simulink model "SteeringWheel"  (R2024b)
settings: configuration reference "STM32H7_Config" (kept outside this file)
libraries: simulink x3
(part 1 of 2)
settings Model: DataDictionary=Master_Dictionary.sldd  EnableAccessToBaseWorkspace=off  Creator=torni  LastModifiedBy=Will
settings ConfigSetRef: SourceName=STM32H7_Config

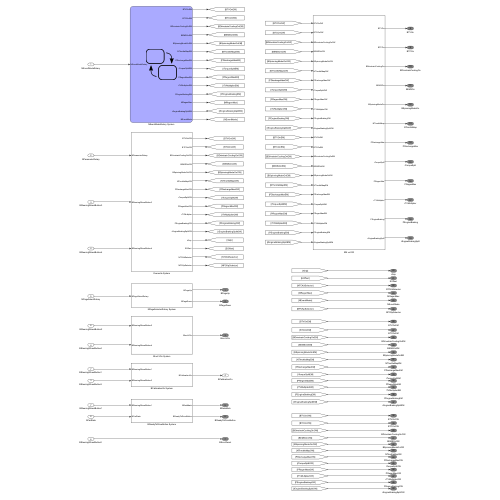
[thumbnail: Simulink's stored preview of the top-level diagram]
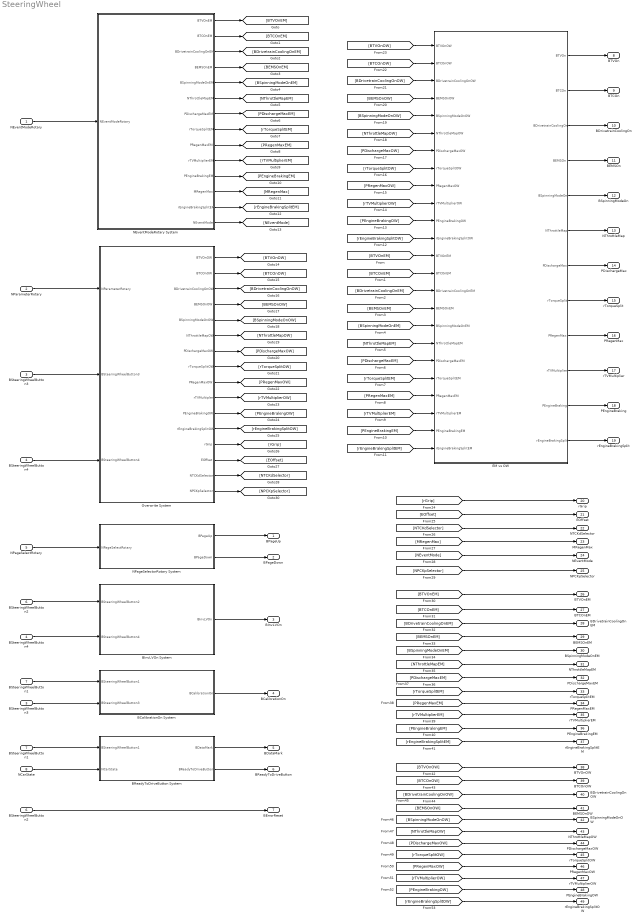
== system SteeringWheel ==
  NEventModeRotary : Inport
  NParameterRotary : Inport  Port=2
  BSteeringWheelButton3 : Inport  Port=3  OutDataTypeStr=boolean
  BSteeringWheelButton4 : Inport  Port=4  OutDataTypeStr=boolean
  NPageSelectRotary : Inport  Port=5
  BSteeringWheelButton2 : Inport  Port=6
  "BSteeringWheelButton1 " : Inport  Port=7
  NCarState : Inport  Port=8
  BCalibrationOn System : Subsystem
  BInvLVOn System : Subsystem
  BReadyToDriveButton System : Subsystem
  BSteeringWheelButton1 : InportShadow  Port=7
  "BSteeringWheelButton2 " : InportShadow  Port=6
  "BSteeringWheelButton3 " : InportShadow  Port=3  OutDataTypeStr=boolean
  "BSteeringWheelButton4 " : InportShadow  Port=4  OutDataTypeStr=boolean
  EM vs OW : Subsystem
  NEventModeRotary System : Stateflow chart  TreatAsAtomicUnit=on
  NPageSelectorRotary System : Subsystem
  Overwrite System : Subsystem
  BPageUp : Outport  VectorParamsAs1DForOutWhenUnconnected=off
  BPageDown : Outport  Port=2  VectorParamsAs1DForOutWhenUnconnected=off
  BInvLVOn : Outport  Port=3  VectorParamsAs1DForOutWhenUnconnected=off
  BCalibrationOn : Outport  Port=4  VectorParamsAs1DForOutWhenUnconnected=off
  BDataMark : Outport  Port=5  VectorParamsAs1DForOutWhenUnconnected=off
  BReadyToDriveButton : Outport  Port=6  VectorParamsAs1DForOutWhenUnconnected=off
  BErrorReset : Outport  Port=7  VectorParamsAs1DForOutWhenUnconnected=off
  BTVOn : Outport  Port=8  VectorParamsAs1DForOutWhenUnconnected=off
  BTCOn : Outport  Port=9  VectorParamsAs1DForOutWhenUnconnected=off
  BDrivetrainCoolingOn : Outport  Port=10  VectorParamsAs1DForOutWhenUnconnected=off
  BEMSOn : Outport  Port=11  VectorParamsAs1DForOutWhenUnconnected=off
  BSpinningModeOn : Outport  Port=12  VectorParamsAs1DForOutWhenUnconnected=off
  NThrottleMap : Outport  Port=13  VectorParamsAs1DForOutWhenUnconnected=off
  PDischargeMax : Outport  Port=14  VectorParamsAs1DForOutWhenUnconnected=off
  rTorqueSplit : Outport  Port=15  VectorParamsAs1DForOutWhenUnconnected=off
  PRegenMax : Outport  Port=16  VectorParamsAs1DForOutWhenUnconnected=off
  rTVMultiplier : Outport  Port=17  VectorParamsAs1DForOutWhenUnconnected=off
  PEngineBraking : Outport  Port=18  VectorParamsAs1DForOutWhenUnconnected=off
  rEngineBrakingSplit : Outport  Port=19  VectorParamsAs1DForOutWhenUnconnected=off
  rGrip : Outport  Port=20  VectorParamsAs1DForOutWhenUnconnected=off
  EOffset : Outport  Port=21  VectorParamsAs1DForOutWhenUnconnected=off
  NTCKdSelector : Outport  Port=22  VectorParamsAs1DForOutWhenUnconnected=off
  MRegenMax : Outport  Port=23  VectorParamsAs1DForOutWhenUnconnected=off
  NEventMode : Outport  Port=24  VectorParamsAs1DForOutWhenUnconnected=off
  NPCKpSelector : Outport  Port=25  VectorParamsAs1DForOutWhenUnconnected=off
  BTVOnEM : Outport  Port=26  OutDataTypeStr=double  VectorParamsAs1DForOutWhenUnconnected=off
  BTCOnEM : Outport  Port=27  OutDataTypeStr=double  VectorParamsAs1DForOutWhenUnconnected=off
  BDrivetrainCoolingOnEM : Outport  Port=28  OutDataTypeStr=double  VectorParamsAs1DForOutWhenUnconnected=off
  BEMSOnEM : Outport  Port=29  OutDataTypeStr=double  VectorParamsAs1DForOutWhenUnconnected=off
  BSpinningModeOnEM : Outport  Port=30  OutDataTypeStr=double  VectorParamsAs1DForOutWhenUnconnected=off
  NThrottleMapEM : Outport  Port=31  OutDataTypeStr=double  VectorParamsAs1DForOutWhenUnconnected=off
  PDischargeMaxEM : Outport  Port=32  OutDataTypeStr=double  VectorParamsAs1DForOutWhenUnconnected=off
  rTorqueSplitEM : Outport  Port=33  OutDataTypeStr=double  VectorParamsAs1DForOutWhenUnconnected=off
  PRegenMaxEM : Outport  Port=34  OutDataTypeStr=double  VectorParamsAs1DForOutWhenUnconnected=off
  rTVMultiplierEM : Outport  Port=35  OutDataTypeStr=double  VectorParamsAs1DForOutWhenUnconnected=off
  PEngineBrakingEM : Outport  Port=36  OutDataTypeStr=double  VectorParamsAs1DForOutWhenUnconnected=off
  rEngineBrakingSplitEM : Outport  Port=37  OutDataTypeStr=double  VectorParamsAs1DForOutWhenUnconnected=off
  BTVOnOW : Outport  Port=38  OutDataTypeStr=double  VectorParamsAs1DForOutWhenUnconnected=off
  BTCOnOW : Outport  Port=39  OutDataTypeStr=double  VectorParamsAs1DForOutWhenUnconnected=off
  BDrivetrainCoolingOnOW : Outport  Port=40  OutDataTypeStr=double  VectorParamsAs1DForOutWhenUnconnected=off
  BEMSOnOW : Outport  Port=41  OutDataTypeStr=double  VectorParamsAs1DForOutWhenUnconnected=off
  BSpinningModeOnOW : Outport  Port=42  OutDataTypeStr=double  VectorParamsAs1DForOutWhenUnconnected=off
  NThrottleMapOW : Outport  Port=43  OutDataTypeStr=double  VectorParamsAs1DForOutWhenUnconnected=off
  PDischargeMaxOW : Outport  Port=44  OutDataTypeStr=double  VectorParamsAs1DForOutWhenUnconnected=off
  rTorqueSplitOW : Outport  Port=45  OutDataTypeStr=double  VectorParamsAs1DForOutWhenUnconnected=off
  PRegenMaxOW : Outport  Port=46  OutDataTypeStr=double  VectorParamsAs1DForOutWhenUnconnected=off
  rTVMultiplierOW : Outport  Port=47  OutDataTypeStr=double  VectorParamsAs1DForOutWhenUnconnected=off
  PEngineBrakingOW : Outport  Port=48  OutDataTypeStr=double  VectorParamsAs1DForOutWhenUnconnected=off
  rEngineBrakingSplitOW : Outport  Port=49  OutDataTypeStr=double  VectorParamsAs1DForOutWhenUnconnected=off
  wires:
  BSteeringWheelButton3/1 -> Overwrite System/2(BSteeringWheelButton3)
  BSteeringWheelButton4/1 -> Overwrite System/3(BSteeringWheelButton4)
  [rEngineBrakingSplitOW] -> rEngineBrakingSplitOW/1
  [PEngineBrakingOW] -> PEngineBrakingOW/1
  [rTVMultiplierOW] -> rTVMultiplierOW/1
  [PRegenMaxOW] -> PRegenMaxOW/1
  [rTorqueSplitOW] -> rTorqueSplitOW/1
  [PDischargeMaxOW] -> PDischargeMaxOW/1
  [NThrottleMapOW] -> NThrottleMapOW/1
  [BSpinningModeOnOW] -> BSpinningModeOnOW/1
  [BEMSOnOW] -> BEMSOnOW/1
  [BDrivetrainCoolingOnOW] -> BDrivetrainCoolingOnOW/1
  [BTCOnOW] -> BTCOnOW/1
  [BTVOnOW] -> BTVOnOW/1
  [rEngineBrakingSplitEM] -> rEngineBrakingSplitEM/1
  [PEngineBrakingEM] -> PEngineBrakingEM/1
  [rTVMultiplierEM] -> rTVMultiplierEM/1
  [PRegenMaxEM] -> PRegenMaxEM/1
  [rTorqueSplitEM] -> rTorqueSplitEM/1
  [PDischargeMaxEM] -> PDischargeMaxEM/1
  [NThrottleMapEM] -> NThrottleMapEM/1
  [BSpinningModeOnEM] -> BSpinningModeOnEM/1
  [BEMSOnEM] -> BEMSOnEM/1
  [BDrivetrainCoolingOnEM] -> BDrivetrainCoolingOnEM/1
  [BTCOnEM] -> BTCOnEM/1
  [BTVOnEM] -> BTVOnEM/1
  [NPCKpSelector] -> NPCKpSelector/1
  [NEventMode] -> NEventMode/1
  [MRegenMax] -> MRegenMax/1
  [NTCKdSelector] -> NTCKdSelector/1
  [EOffset] -> EOffset/1
  [rGrip] -> rGrip/1
  EM vs OW/12(rEngineBrakingSplit) -> rEngineBrakingSplit/1
  EM vs OW/11(PEngineBraking) -> PEngineBraking/1
  EM vs OW/10(rTVMultiplier) -> rTVMultiplier/1
  EM vs OW/9(PRegenMax) -> PRegenMax/1
  EM vs OW/8(rTorqueSplit) -> rTorqueSplit/1
  EM vs OW/7(PDischargeMax) -> PDischargeMax/1
  EM vs OW/6(NThrottleMap) -> NThrottleMap/1
  EM vs OW/5(BSpinningModeOn) -> BSpinningModeOn/1
  EM vs OW/4(BEMSOn) -> BEMSOn/1
  EM vs OW/3(BDrivetrainCoolingOn) -> BDrivetrainCoolingOn/1
  EM vs OW/2(BTCOn) -> BTCOn/1
  EM vs OW/1(BTVOn) -> BTVOn/1
  NEventModeRotary System/14(NEventMode) -> [NEventMode]
  NEventModeRotary System/13(rEngineBrakingSplitEM) -> [rEngineBrakingSplitEM]
  NEventModeRotary System/12(MRegenMax) -> [MRegenMax]
  NEventModeRotary System/11(PEngineBrakingEM) -> [PEngineBrakingEM]
  NEventModeRotary System/10(rTVMultiplierEM) -> [rTVMultiplierEM]
  NEventModeRotary System/9(PRegenMaxEM) -> [PRegenMaxEM]
  NEventModeRotary System/8(rTorqueSplitEM) -> [rTorqueSplitEM]
  NEventModeRotary System/7(PDischargeMaxEM) -> [PDischargeMaxEM]
  NEventModeRotary System/6(NThrottleMapEM) -> [NThrottleMapEM]
  NEventModeRotary System/5(BSpinningModeOnEM) -> [BSpinningModeOnEM]
  NEventModeRotary System/4(BEMSOnEM) -> [BEMSOnEM]
  NEventModeRotary System/3(BDrivetrainCoolingOnEM) -> [BDrivetrainCoolingOnEM]
  NEventModeRotary System/2(BTCOnEM) -> [BTCOnEM]
  NEventModeRotary System/1(BTVOnEM) -> [BTVOnEM]
  NEventModeRotary/1 -> NEventModeRotary System/1(NEventModeRotary)
  Overwrite System/15(NTCKdSelector) -> [NTCKdSelector]
  Overwrite System/14("EOffset ") -> [EOffset]
  Overwrite System/13("rGrip ") -> [rGrip]
  Overwrite System/12(rEngineBrakingSplitOW) -> [rEngineBrakingSplitOW]
  Overwrite System/11(PEngineBrakingOW) -> [PEngineBrakingOW]
  Overwrite System/10(rTVMultipler) -> [rTVMultiplierOW]
  Overwrite System/9(PRegenMaxOW) -> [PRegenMaxOW]
  Overwrite System/8(rTorqueSplitOW) -> [rTorqueSplitOW]
  Overwrite System/7(PDischargeMaxOW) -> [PDischargeMaxOW]
  Overwrite System/6(NThrottleMapOW) -> [NThrottleMapOW]
  Overwrite System/5(BSpinningModeOnOW) -> [BSpinningModeOnOW]
  Overwrite System/4(BEMSOnOW) -> [BEMSOnOW]
  Overwrite System/3(BDrivetrainCoolingOnOW) -> [BDrivetrainCoolingOnOW]
  Overwrite System/2(BTCOnOW) -> [BTCOnOW]
  Overwrite System/1(BTVOnOW) -> [BTVOnOW]
  Overwrite System/16(NPCKpSelector) -> [NPCKpSelector]
  NParameterRotary/1 -> Overwrite System/1(NParameterRotary)
  NPageSelectRotary/1 -> NPageSelectorRotary System/1(NPageSelectRotary)
  NPageSelectorRotary System/1(BPageUp) -> BPageUp/1
  NPageSelectorRotary System/2(BPageDown) -> BPageDown/1
  BSteeringWheelButton2/1 -> BInvLVOn System/1(BSteeringWheelButton2)
  "BSteeringWheelButton4 "/1 -> BInvLVOn System/2(BSteeringWheelButton4)
  BInvLVOn System/1(BInvLVOn) -> BInvLVOn/1
  "BSteeringWheelButton1 "/1 -> BCalibrationOn System/1(BSteeringWheelButton1)
  "BSteeringWheelButton3 "/1 -> BCalibrationOn System/2("BSteeringWheelButton3 ")
  BCalibrationOn System/1(BCalibrationOn) -> BCalibrationOn/1
  BReadyToDriveButton System/1(BDataMark) -> BDataMark/1
  BReadyToDriveButton System/2(BReadyToDriveButton) -> BReadyToDriveButton/1
  BSteeringWheelButton1/1 -> BReadyToDriveButton System/1(BSteeringWheelButton1)
  NCarState/1 -> BReadyToDriveButton System/2(NCarState)
  "BSteeringWheelButton2 "/1 -> BErrorReset/1
  [BTVOnOW] -> EM vs OW/1(BTVOnOW)
  [BTCOnOW] -> EM vs OW/2(BTCOnOW)
  [BDrivetrainCoolingOnOW] -> EM vs OW/3(BDrivetrainCoolingOnOW)
  [BEMSOnOW] -> EM vs OW/4(BEMSOnOW)
  [BSpinningModeOnOW] -> EM vs OW/5(BSpinningModeOnOW)
  [NThrottleMapOW] -> EM vs OW/6(NThrottleMapOW)
  [PDischargeMaxOW] -> EM vs OW/7(PDischargeMaxOW)
  [rTorqueSplitOW] -> EM vs OW/8(rTorqueSplitOW)
  [PRegenMaxOW] -> EM vs OW/9(PRegenMaxOW)
  [rTVMultiplierOW] -> EM vs OW/10(rTVMultiplierOW)
  [PEngineBrakingOW] -> EM vs OW/11(PEngineBrakingOW)
  [rEngineBrakingSplitOW] -> EM vs OW/12(rEngineBrakingSplitOW)
  [BTVOnEM] -> EM vs OW/13(BTVOnEM)
  [BTCOnEM] -> EM vs OW/14(BTCOnEM)
  [BDrivetrainCoolingOnEM] -> EM vs OW/15(BDrivetrainCoolingOnEM)
  [BEMSOnEM] -> EM vs OW/16(BEMSOnEM)
  [BSpinningModeOnEM] -> EM vs OW/17(BSpinningModeOnEM)
  [NThrottleMapEM] -> EM vs OW/18(NThrottleMapEM)
  [PDischargeMaxEM] -> EM vs OW/19(PDischargeMaxEM)
  [rTorqueSplitEM] -> EM vs OW/20(rTorqueSplitEM)
  [PRegenMaxEM] -> EM vs OW/21(PRegenMaxEM)
  [rTVMultiplierEM] -> EM vs OW/22(rTVMultiplierEM)
  [PEngineBrakingEM] -> EM vs OW/23(PEngineBrakingEM)
  [rEngineBrakingSplitEM] -> EM vs OW/24(rEngineBrakingSplitEM)

== system SteeringWheel/BCalibrationOn System ==
  BSteeringWheelButton1 : Inport
  "BSteeringWheelButton3 " : Inport  Port=2
  AND : Logic  AllPortsSameDT=off  OutDataTypeStr=boolean
  BCalibrationOn : Outport  VectorParamsAs1DForOutWhenUnconnected=off
  wires:
  BSteeringWheelButton1/1 -> AND/1
  AND/1 -> BCalibrationOn/1
  "BSteeringWheelButton3 "/1 -> AND/2

== system SteeringWheel/BInvLVOn System ==
  BSteeringWheelButton2 : Inport
  BSteeringWheelButton4 : Inport  Port=2
  AND1 : Logic  Operator=NAND  AllPortsSameDT=off  OutDataTypeStr=boolean
  BInvLVOn : Outport  VectorParamsAs1DForOutWhenUnconnected=off
  wires:
  AND1/1 -> BInvLVOn/1
  BSteeringWheelButton2/1 -> AND1/1
  BSteeringWheelButton4/1 -> AND1/2

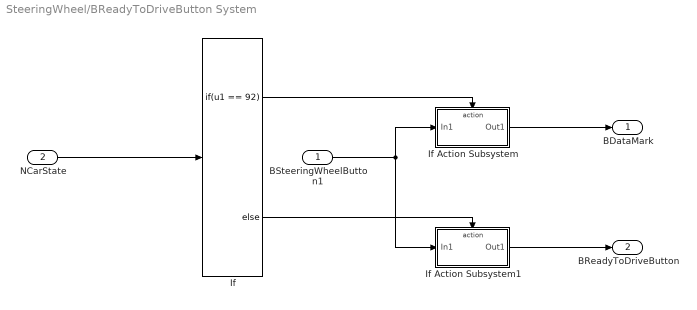
== system SteeringWheel/BReadyToDriveButton System ==
  BSteeringWheelButton1 : Inport
  NCarState : Inport  Port=2
  If : If  IfExpression=u1 == 92
  If Action Subsystem : Subsystem  TreatAsAtomicUnit=on
  If Action Subsystem1 : Subsystem  TreatAsAtomicUnit=on
  BDataMark : Outport  VectorParamsAs1DForOutWhenUnconnected=off
  BReadyToDriveButton : Outport  Port=2  VectorParamsAs1DForOutWhenUnconnected=off
  wires:
  If/2 -> If Action Subsystem1/Action
  If Action Subsystem/1(Out1) -> BDataMark/1
  If Action Subsystem1/1(Out1) -> BReadyToDriveButton/1
  BSteeringWheelButton1/1 -> If Action Subsystem1/1(In1), If Action Subsystem/1(In1)
  NCarState/1 -> If/1
  If/1 -> If Action Subsystem/Action

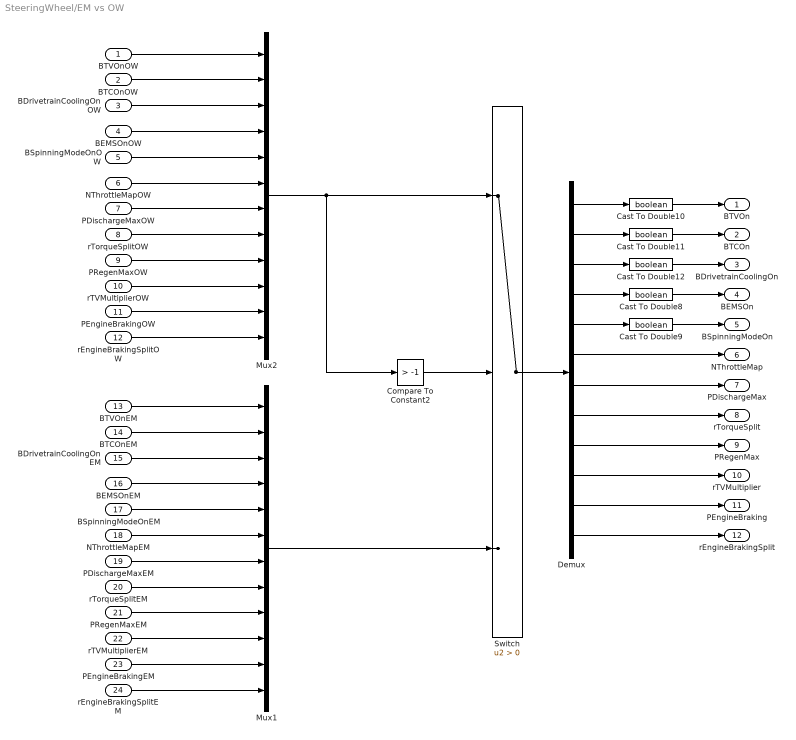
== system SteeringWheel/EM vs OW ==
  BTVOnOW : Inport
  BTCOnOW : Inport  Port=2
  BDrivetrainCoolingOnOW : Inport  Port=3
  BEMSOnOW : Inport  Port=4
  BSpinningModeOnOW : Inport  Port=5
  NThrottleMapOW : Inport  Port=6
  PDischargeMaxOW : Inport  Port=7
  rTorqueSplitOW : Inport  Port=8
  PRegenMaxOW : Inport  Port=9
  rTVMultiplierOW : Inport  Port=10
  PEngineBrakingOW : Inport  Port=11
  rEngineBrakingSplitOW : Inport  Port=12
  BTVOnEM : Inport  Port=13
  BTCOnEM : Inport  Port=14
  BDrivetrainCoolingOnEM : Inport  Port=15
  BEMSOnEM : Inport  Port=16
  BSpinningModeOnEM : Inport  Port=17
  NThrottleMapEM : Inport  Port=18
  PDischargeMaxEM : Inport  Port=19
  rTorqueSplitEM : Inport  Port=20
  PRegenMaxEM : Inport  Port=21
  rTVMultiplierEM : Inport  Port=22
  PEngineBrakingEM : Inport  Port=23
  rEngineBrakingSplitEM : Inport  Port=24
  Cast To Double{8..12} (5 alike) : DataTypeConversion  OutDataTypeStr=boolean  SaturateOnIntegerOverflow=off  RndMeth=Floor
  Compare To Constant2 : simulink/Logic and Bit Operations/Compare To Constant  relop=>  const=-1  OutDataTypeStr=boolean
  Demux : Demux  Outputs=12
  Mux1 : Mux  Inputs=12
  Mux2 : Mux  Inputs=12
  Switch : Switch  Criteria=u2 > Threshold  OutDataTypeStr=double  SaturateOnIntegerOverflow=off  InputSameDT=off
  BTVOn : Outport  VectorParamsAs1DForOutWhenUnconnected=off
  BTCOn : Outport  Port=2  VectorParamsAs1DForOutWhenUnconnected=off
  BDrivetrainCoolingOn : Outport  Port=3  VectorParamsAs1DForOutWhenUnconnected=off
  BEMSOn : Outport  Port=4  VectorParamsAs1DForOutWhenUnconnected=off
  BSpinningModeOn : Outport  Port=5  VectorParamsAs1DForOutWhenUnconnected=off
  NThrottleMap : Outport  Port=6  VectorParamsAs1DForOutWhenUnconnected=off
  PDischargeMax : Outport  Port=7  VectorParamsAs1DForOutWhenUnconnected=off
  rTorqueSplit : Outport  Port=8  VectorParamsAs1DForOutWhenUnconnected=off
  PRegenMax : Outport  Port=9  VectorParamsAs1DForOutWhenUnconnected=off
  rTVMultiplier : Outport  Port=10  VectorParamsAs1DForOutWhenUnconnected=off
  PEngineBraking : Outport  Port=11  VectorParamsAs1DForOutWhenUnconnected=off
  rEngineBrakingSplit : Outport  Port=12  VectorParamsAs1DForOutWhenUnconnected=off
  wires:
  Demux/4 -> Cast To Double8/1
  Demux/5 -> Cast To Double9/1
  Demux/11 -> PEngineBraking/1
  Demux/1 -> Cast To Double10/1
  BSpinningModeOnOW/1 -> Mux2/5
  Demux/6 -> NThrottleMap/1
  rEngineBrakingSplitOW/1 -> Mux2/12
  Cast To Double9/1 -> BSpinningModeOn/1
  BEMSOnOW/1 -> Mux2/4
  Mux2/1 -> Compare To Constant2/1, Switch/1
  Compare To Constant2/1 -> Switch/2
  PRegenMaxEM/1 -> Mux1/9
  PEngineBrakingOW/1 -> Mux2/11
  Switch/1 -> Demux/1
  Mux1/1 -> Switch/3
  BTCOnEM/1 -> Mux1/2
  Demux/2 -> Cast To Double11/1
  Demux/3 -> Cast To Double12/1
  Demux/10 -> rTVMultiplier/1
  PRegenMaxOW/1 -> Mux2/9
  BTCOnOW/1 -> Mux2/2
  rTVMultiplierOW/1 -> Mux2/10
  rEngineBrakingSplitEM/1 -> Mux1/12
  BTVOnEM/1 -> Mux1/1
  BEMSOnEM/1 -> Mux1/4
  Demux/12 -> rEngineBrakingSplit/1
  BDrivetrainCoolingOnEM/1 -> Mux1/3
  Demux/7 -> PDischargeMax/1
  rTVMultiplierEM/1 -> Mux1/10
  BDrivetrainCoolingOnOW/1 -> Mux2/3
  Demux/9 -> PRegenMax/1
  Cast To Double8/1 -> BEMSOn/1
  NThrottleMapOW/1 -> Mux2/6
  rTorqueSplitOW/1 -> Mux2/8
  Cast To Double12/1 -> BDrivetrainCoolingOn/1
  Demux/8 -> rTorqueSplit/1
  NThrottleMapEM/1 -> Mux1/6
  PDischargeMaxOW/1 -> Mux2/7
  rTorqueSplitEM/1 -> Mux1/8
  Cast To Double11/1 -> BTCOn/1
  PDischargeMaxEM/1 -> Mux1/7
  BSpinningModeOnEM/1 -> Mux1/5
  Cast To Double10/1 -> BTVOn/1
  PEngineBrakingEM/1 -> Mux1/11
  BTVOnOW/1 -> Mux2/1

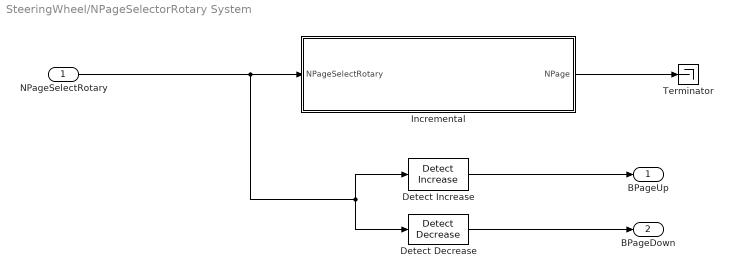
== system SteeringWheel/NPageSelectorRotary System ==
  NPageSelectRotary : Inport
  Detect Decrease : simulink/Logic and Bit Operations/Detect Decrease  vinit=0.0  OutDataTypeStr=boolean
  Detect Increase : simulink/Logic and Bit Operations/Detect Increase  vinit=0.0  OutDataTypeStr=boolean
  Incremental : Stateflow chart  TreatAsAtomicUnit=on
  Terminator : Terminator
  BPageUp : Outport  VectorParamsAs1DForOutWhenUnconnected=off
  BPageDown : Outport  Port=2  VectorParamsAs1DForOutWhenUnconnected=off
  wires:
  NPageSelectRotary/1 -> Incremental/1(NPageSelectRotary), Detect Decrease/1, Detect Increase/1
  Detect Decrease/1 -> BPageDown/1
  Detect Increase/1 -> BPageUp/1
  Incremental/1(NPage) -> Terminator/1

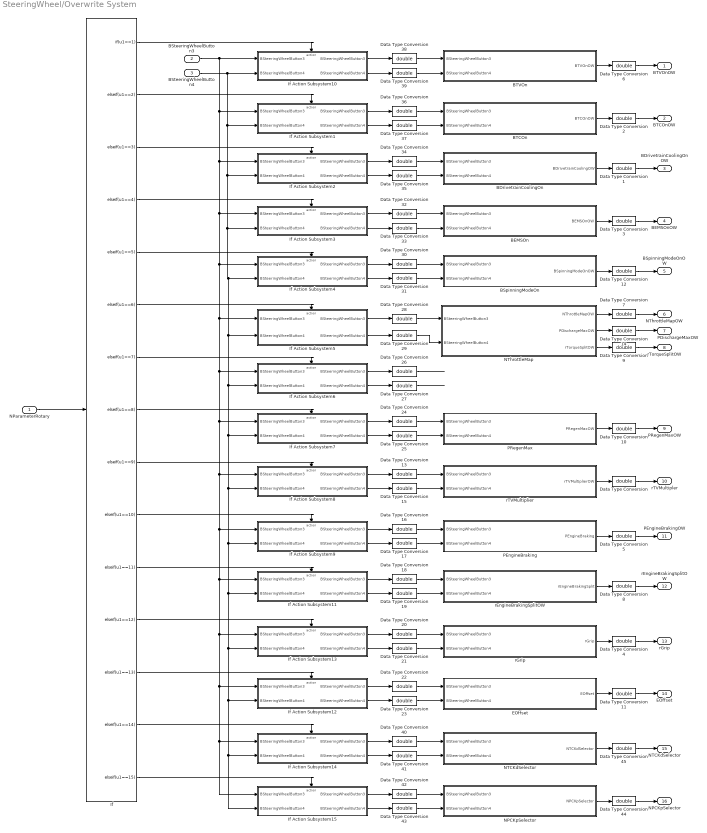
== system SteeringWheel/Overwrite System ==
  NParameterRotary : Inport  OutDataTypeStr=double
  BSteeringWheelButton3 : Inport  Port=2  OutDataTypeStr=boolean
  BSteeringWheelButton4 : Inport  Port=3  OutDataTypeStr=boolean
  BDrivetrainCoolingOn : Stateflow chart  TreatAsAtomicUnit=on
  BEMSOn : Stateflow chart  TreatAsAtomicUnit=on
  BSpinningModeOn : Stateflow chart  TreatAsAtomicUnit=on
  BTCOn : Stateflow chart  TreatAsAtomicUnit=on
  BTVOn : Stateflow chart  TreatAsAtomicUnit=on
  Data Type Conversion{,1..45} (46 alike) : DataTypeConversion  OutDataTypeStr=double  SaturateOnIntegerOverflow=off  RndMeth=Floor
  EOffset : Stateflow chart  TreatAsAtomicUnit=on
  If : If  IfExpression=u1==1  ElseIfExpressions=u1==2, u1==3, u1==4, u1==5, u1==6, u1==7, u1==8, u1==9, u1==10, u1==11, u1==12, u1==13, u1==14, u1==15  ShowElse=off
  If Action Subsystem1 : Subsystem  TreatAsAtomicUnit=on
  If Action Subsystem10 : Subsystem  TreatAsAtomicUnit=on
  If Action Subsystem11 : Subsystem  TreatAsAtomicUnit=on
  If Action Subsystem12 : Subsystem  TreatAsAtomicUnit=on
  If Action Subsystem13 : Subsystem  TreatAsAtomicUnit=on
  If Action Subsystem14 : Subsystem  TreatAsAtomicUnit=on
  If Action Subsystem15 : Subsystem  TreatAsAtomicUnit=on
  If Action Subsystem2 : Subsystem  TreatAsAtomicUnit=on
  If Action Subsystem3 : Subsystem  TreatAsAtomicUnit=on
  If Action Subsystem4 : Subsystem  TreatAsAtomicUnit=on
  If Action Subsystem5 : Subsystem  TreatAsAtomicUnit=on
  If Action Subsystem6 : Subsystem  TreatAsAtomicUnit=on
  If Action Subsystem7 : Subsystem  TreatAsAtomicUnit=on
  If Action Subsystem8 : Subsystem  TreatAsAtomicUnit=on
  If Action Subsystem9 : Subsystem  TreatAsAtomicUnit=on
  "NPCKpSelector " : Stateflow chart  TreatAsAtomicUnit=on
  "NTCKdSelector " : Stateflow chart  TreatAsAtomicUnit=on
  NThrottleMap : Stateflow chart  TreatAsAtomicUnit=on
  PEngineBraking : Stateflow chart  TreatAsAtomicUnit=on
  PRegenMax : Stateflow chart  TreatAsAtomicUnit=on
  "rEngineBrakingSplitOW " : Stateflow chart  TreatAsAtomicUnit=on
  rGrip : Stateflow chart  TreatAsAtomicUnit=on
  rTVMultiplier : Stateflow chart  TreatAsAtomicUnit=on
  BTVOnOW : Outport  OutDataTypeStr=double  VectorParamsAs1DForOutWhenUnconnected=off
  BTCOnOW : Outport  Port=2  OutDataTypeStr=double  VectorParamsAs1DForOutWhenUnconnected=off
  BDrivetrainCoolingOnOW : Outport  Port=3  OutDataTypeStr=double  VectorParamsAs1DForOutWhenUnconnected=off
  BEMSOnOW : Outport  Port=4  OutDataTypeStr=double  VectorParamsAs1DForOutWhenUnconnected=off
  BSpinningModeOnOW : Outport  Port=5  OutDataTypeStr=double  VectorParamsAs1DForOutWhenUnconnected=off
  NThrottleMapOW : Outport  Port=6  OutDataTypeStr=double  VectorParamsAs1DForOutWhenUnconnected=off
  PDischargeMaxOW : Outport  Port=7  OutDataTypeStr=double  VectorParamsAs1DForOutWhenUnconnected=off
  rTorqueSplitOW : Outport  Port=8  OutDataTypeStr=double  VectorParamsAs1DForOutWhenUnconnected=off
  PRegenMaxOW : Outport  Port=9  OutDataTypeStr=double  VectorParamsAs1DForOutWhenUnconnected=off
  rTVMultipler : Outport  Port=10  OutDataTypeStr=double  VectorParamsAs1DForOutWhenUnconnected=off
  PEngineBrakingOW : Outport  Port=11  OutDataTypeStr=double  VectorParamsAs1DForOutWhenUnconnected=off
  rEngineBrakingSplitOW : Outport  Port=12  OutDataTypeStr=double  VectorParamsAs1DForOutWhenUnconnected=off
  "rGrip " : Outport  Port=13  OutDataTypeStr=double  VectorParamsAs1DForOutWhenUnconnected=off
  "EOffset " : Outport  Port=14  OutDataTypeStr=double  VectorParamsAs1DForOutWhenUnconnected=off
  NTCKdSelector : Outport  Port=15  OutDataTypeStr=double  VectorParamsAs1DForOutWhenUnconnected=off
  NPCKpSelector : Outport  Port=16  OutDataTypeStr=double  VectorParamsAs1DForOutWhenUnconnected=off
  wires:
  If/5 -> If Action Subsystem4/Action
  Data Type Conversion45/1 -> NTCKdSelector/1
  If Action Subsystem3/1(BSteeringWheelButton3) -> Data Type Conversion32/1
  "rEngineBrakingSplitOW "/1(rEngineBrakingSplit) -> Data Type Conversion8/1
  Data Type Conversion30/1 -> BSpinningModeOn/1(BSteeringWheelButton3)
  Data Type Conversion6/1 -> BTVOnOW/1
  Data Type Conversion40/1 -> "NTCKdSelector "/1(BSteeringWheelButton3)
  Data Type Conversion1/1 -> BDrivetrainCoolingOnOW/1
  Data Type Conversion19/1 -> "rEngineBrakingSplitOW "/2(BSteeringWheelButton4)
  If Action Subsystem7/2(BSteeringWheelButton4) -> Data Type Conversion25/1
  If/14 -> If Action Subsystem14/Action
  Data Type Conversion32/1 -> BEMSOn/1(BSteeringWheelButton3)
  Data Type Conversion39/1 -> BTVOn/2(BSteeringWheelButton4)
  Data Type Conversion8/1 -> rEngineBrakingSplitOW/1
  Data Type Conversion34/1 -> BDrivetrainCoolingOn/1(BSteeringWheelButton3)
  rTVMultiplier/1(rTVMultiplierOW) -> Data Type Conversion/1
  Data Type Conversion23/1 -> EOffset/2(BSteeringWheelButton4)
  Data Type Conversion43/1 -> "NPCKpSelector "/2(BSteeringWheelButton4)
  If Action Subsystem2/2(BSteeringWheelButton4) -> Data Type Conversion35/1
  Data Type Conversion15/1 -> rTVMultiplier/2(BSteeringWheelButton4)
  If Action Subsystem9/2(BSteeringWheelButton4) -> Data Type Conversion17/1
  Data Type Conversion31/1 -> BSpinningModeOn/2(BSteeringWheelButton4)
  Data Type Conversion5/1 -> PEngineBrakingOW/1
  NThrottleMap/1(NThrottleMapOW) -> Data Type Conversion7/1
  If/8 -> If Action Subsystem7/Action
  Data Type Conversion4/1 -> "rGrip "/1
  If Action Subsystem5/1(BSteeringWheelButton3) -> Data Type Conversion28/1
  If/11 -> If Action Subsystem11/Action
  If Action Subsystem14/1(BSteeringWheelButton3) -> Data Type Conversion40/1
  NThrottleMap/3(rTorqueSplitOW) -> Data Type Conversion9/1
  BTCOn/1(BTCOnOW) -> Data Type Conversion2/1
  If Action Subsystem14/2(BSteeringWheelButton4) -> Data Type Conversion41/1
  Data Type Conversion42/1 -> "NPCKpSelector "/1(BSteeringWheelButton3)
  Data Type Conversion35/1 -> BDrivetrainCoolingOn/2(BSteeringWheelButton4)
  Data Type Conversion36/1 -> BTCOn/1(BSteeringWheelButton3)
  If Action Subsystem8/1(BSteeringWheelButton3) -> Data Type Conversion13/1
  Data Type Conversion29/1 -> NThrottleMap/2(BSteeringWheelButton4)
  Data Type Conversion37/1 -> BTCOn/2(BSteeringWheelButton4)
  Data Type Conversion18/1 -> "rEngineBrakingSplitOW "/1(BSteeringWheelButton3)
  If/15 -> If Action Subsystem15/Action
  BSteeringWheelButton4/1 -> If Action Subsystem8/2("BSteeringWheelButton4  "), If Action Subsystem9/2("BSteeringWheelButton4  "), If Action Subsystem11/2("BSteeringWheelButton4  "), If Action Subsystem13/2("BSteeringWheelButton4  "), If Action Subsystem15/2("BSteeringWheelButton4  "), If Action Subsystem14/2("BSteeringWheelButton4  "), If Action Subsystem12/2("BSteeringWheelButton4  "), If Action Subsystem7/2("BSteeringWheelButton4  "), If Action Subsystem6/2("BSteeringWheelButton4  "), If Action Subsystem5/2("BSteeringWheelButton4  "), If Action Subsystem4/2("BSteeringWheelButton4  "), If Action Subsystem3/2("BSteeringWheelButton4  "), If Action Subsystem2/2("BSteeringWheelButton4  "), If Action Subsystem1/2("BSteeringWheelButton4  "), If Action Subsystem10/2("BSteeringWheelButton4  ")
  "NPCKpSelector "/1(NPCKpSelector) -> Data Type Conversion44/1
  If Action Subsystem1/2(BSteeringWheelButton4) -> Data Type Conversion37/1
  Data Type Conversion9/1 -> rTorqueSplitOW/1
  Data Type Conversion11/1 -> "EOffset "/1
  Data Type Conversion20/1 -> rGrip/1(BSteeringWheelButton3)
  Data Type Conversion28/1 -> NThrottleMap/1(BSteeringWheelButton3)
  NParameterRotary/1 -> If/1
  If Action Subsystem3/2(BSteeringWheelButton4) -> Data Type Conversion33/1
  Data Type Conversion24/1 -> PRegenMax/1(BSteeringWheelButton3)
  Data Type Conversion27/1 -> ?
  Data Type Conversion21/1 -> rGrip/2(BSteeringWheelButton4)
  BDrivetrainCoolingOn/1(BDrivetrainCoolingOW) -> Data Type Conversion1/1
  If Action Subsystem13/1(BSteeringWheelButton3) -> Data Type Conversion20/1
  If Action Subsystem8/2(BSteeringWheelButton4) -> Data Type Conversion15/1
  Data Type Conversion26/1 -> ?
  Data Type Conversion25/1 -> PRegenMax/2(BSteeringWheelButton4)
  If Action Subsystem6/1(BSteeringWheelButton3) -> Data Type Conversion26/1
  Data Type Conversion13/1 -> rTVMultiplier/1(BSteeringWheelButton3)
  BSteeringWheelButton3/1 -> If Action Subsystem10/1("BSteeringWheelButton3  "), If Action Subsystem8/1("BSteeringWheelButton3  "), If Action Subsystem9/1("BSteeringWheelButton3  "), If Action Subsystem11/1("BSteeringWheelButton3  "), If Action Subsystem13/1("BSteeringWheelButton3  "), If Action Subsystem15/1("BSteeringWheelButton3  "), If Action Subsystem14/1("BSteeringWheelButton3  "), If Action Subsystem12/1("BSteeringWheelButton3  "), If Action Subsystem7/1("BSteeringWheelButton3  "), If Action Subsystem6/1("BSteeringWheelButton3  "), If Action Subsystem5/1("BSteeringWheelButton3  "), If Action Subsystem4/1("BSteeringWheelButton3  "), If Action Subsystem3/1("BSteeringWheelButton3  "), If Action Subsystem2/1("BSteeringWheelButton3  "), If Action Subsystem1/1("BSteeringWheelButton3  ")
  If Action Subsystem12/2(BSteeringWheelButton4) -> Data Type Conversion23/1
  "NTCKdSelector "/1(NTCKdSelector) -> Data Type Conversion45/1
  If Action Subsystem10/1(BSteeringWheelButton3) -> Data Type Conversion38/1
  If Action Subsystem11/1(BSteeringWheelButton3) -> Data Type Conversion18/1
  If Action Subsystem15/1(BSteeringWheelButton3) -> Data Type Conversion42/1
  NThrottleMap/2(PDischargeMaxOW) -> Data Type Conversion14/1
  Data Type Conversion12/1 -> BSpinningModeOnOW/1
  If/1 -> If Action Subsystem10/Action
  BSpinningModeOn/1(BSpinningModeOnOW) -> Data Type Conversion12/1
  Data Type Conversion17/1 -> PEngineBraking/2(BSteeringWheelButton4)
  If Action Subsystem6/2(BSteeringWheelButton4) -> Data Type Conversion27/1
  If Action Subsystem11/2(BSteeringWheelButton4) -> Data Type Conversion19/1
  PEngineBraking/1(PEngineBraking) -> Data Type Conversion5/1
  rGrip/1(rGrip) -> Data Type Conversion4/1
  If Action Subsystem10/2(BSteeringWheelButton4) -> Data Type Conversion39/1
  If Action Subsystem4/2(BSteeringWheelButton4) -> Data Type Conversion31/1
  If Action Subsystem9/1(BSteeringWheelButton3) -> Data Type Conversion16/1
  If/9 -> If Action Subsystem8/Action
  BTVOn/1(BTVOnOW) -> Data Type Conversion6/1
  If Action Subsystem4/1(BSteeringWheelButton3) -> Data Type Conversion30/1
  If Action Subsystem13/2(BSteeringWheelButton4) -> Data Type Conversion21/1
  Data Type Conversion7/1 -> NThrottleMapOW/1
  BEMSOn/1(BEMSOnOW) -> Data Type Conversion3/1
  If/3 -> If Action Subsystem2/Action
  Data Type Conversion2/1 -> BTCOnOW/1
  If/13 -> If Action Subsystem12/Action
  If Action Subsystem12/1(BSteeringWheelButton3) -> Data Type Conversion22/1
  If/6 -> If Action Subsystem5/Action
  Data Type Conversion/1 -> rTVMultipler/1
  Data Type Conversion33/1 -> BEMSOn/2(BSteeringWheelButton4)
  If/12 -> If Action Subsystem13/Action
  Data Type Conversion16/1 -> PEngineBraking/1(BSteeringWheelButton3)
  Data Type Conversion14/1 -> PDischargeMaxOW/1
  Data Type Conversion44/1 -> NPCKpSelector/1
  If Action Subsystem2/1(BSteeringWheelButton3) -> Data Type Conversion34/1
  PRegenMax/1(PRegenMaxOW) -> Data Type Conversion10/1
  Data Type Conversion38/1 -> BTVOn/1(BSteeringWheelButton3)
  If/2 -> If Action Subsystem1/Action
  If Action Subsystem1/1(BSteeringWheelButton3) -> Data Type Conversion36/1
  If Action Subsystem15/2(BSteeringWheelButton4) -> Data Type Conversion43/1
  If Action Subsystem5/2(BSteeringWheelButton4) -> Data Type Conversion29/1
  Data Type Conversion10/1 -> PRegenMaxOW/1
  Data Type Conversion3/1 -> BEMSOnOW/1
  If Action Subsystem7/1(BSteeringWheelButton3) -> Data Type Conversion24/1
  Data Type Conversion22/1 -> EOffset/1(BSteeringWheelButton3)
  If/10 -> If Action Subsystem9/Action
  EOffset/1(EOffset) -> Data Type Conversion11/1
  If/7 -> If Action Subsystem6/Action
  If/4 -> If Action Subsystem3/Action
  Data Type Conversion41/1 -> "NTCKdSelector "/2(BSteeringWheelButton4)

== system SteeringWheel/BReadyToDriveButton System/If Action Subsystem ==
  In1 : Inport
  Action Port : ActionPort  ActionPortLabel=if(u1 == 92)
  Out1 : Outport  VectorParamsAs1DForOutWhenUnconnected=off
  wires:
  In1/1 -> Out1/1

== system SteeringWheel/BReadyToDriveButton System/If Action Subsystem1 ==
  In1 : Inport
  Action Port : ActionPort  ActionPortLabel=else
  Out1 : Outport  VectorParamsAs1DForOutWhenUnconnected=off
  wires:
  In1/1 -> Out1/1

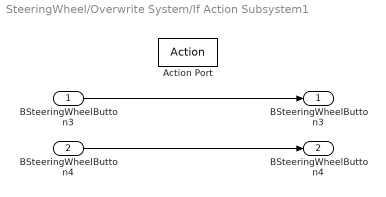
== system SteeringWheel/Overwrite System/If Action Subsystem1 ==
  "BSteeringWheelButton3  " : Inport  OutDataTypeStr=boolean
  "BSteeringWheelButton4  " : Inport  Port=2  OutDataTypeStr=boolean
  Action Port : ActionPort  ActionPortLabel=elseif(u1==2)
  BSteeringWheelButton3 : Outport  OutDataTypeStr=boolean  VectorParamsAs1DForOutWhenUnconnected=off
  BSteeringWheelButton4 : Outport  Port=2  OutDataTypeStr=boolean  VectorParamsAs1DForOutWhenUnconnected=off
  wires:
  "BSteeringWheelButton4  "/1 -> BSteeringWheelButton4/1
  "BSteeringWheelButton3  "/1 -> BSteeringWheelButton3/1

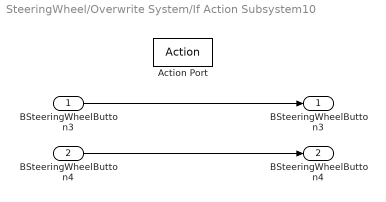
== system SteeringWheel/Overwrite System/If Action Subsystem10 ==
  "BSteeringWheelButton3  " : Inport  OutDataTypeStr=boolean
  "BSteeringWheelButton4  " : Inport  Port=2  OutDataTypeStr=boolean
  Action Port : ActionPort  ActionPortLabel=if(u1==1)
  BSteeringWheelButton3 : Outport  OutDataTypeStr=boolean  VectorParamsAs1DForOutWhenUnconnected=off
  BSteeringWheelButton4 : Outport  Port=2  OutDataTypeStr=boolean  VectorParamsAs1DForOutWhenUnconnected=off
  wires:
  "BSteeringWheelButton4  "/1 -> BSteeringWheelButton4/1
  "BSteeringWheelButton3  "/1 -> BSteeringWheelButton3/1

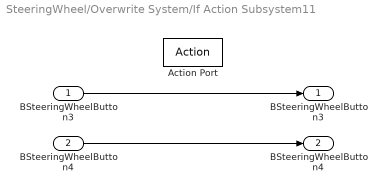
== system SteeringWheel/Overwrite System/If Action Subsystem11 ==
  "BSteeringWheelButton3  " : Inport  OutDataTypeStr=boolean
  "BSteeringWheelButton4  " : Inport  Port=2  OutDataTypeStr=boolean
  Action Port : ActionPort  ActionPortLabel=elseif( u1==11)
  BSteeringWheelButton3 : Outport  OutDataTypeStr=boolean  VectorParamsAs1DForOutWhenUnconnected=off
  BSteeringWheelButton4 : Outport  Port=2  OutDataTypeStr=boolean  VectorParamsAs1DForOutWhenUnconnected=off
  wires:
  "BSteeringWheelButton3  "/1 -> BSteeringWheelButton3/1
  "BSteeringWheelButton4  "/1 -> BSteeringWheelButton4/1

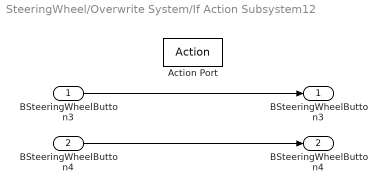
== system SteeringWheel/Overwrite System/If Action Subsystem12 ==
  "BSteeringWheelButton3  " : Inport  OutDataTypeStr=boolean
  "BSteeringWheelButton4  " : Inport  Port=2  OutDataTypeStr=boolean
  Action Port : ActionPort  ActionPortLabel=elseif( u1==13)
  BSteeringWheelButton3 : Outport  OutDataTypeStr=boolean  VectorParamsAs1DForOutWhenUnconnected=off
  BSteeringWheelButton4 : Outport  Port=2  OutDataTypeStr=boolean  VectorParamsAs1DForOutWhenUnconnected=off
  wires:
  "BSteeringWheelButton3  "/1 -> BSteeringWheelButton3/1
  "BSteeringWheelButton4  "/1 -> BSteeringWheelButton4/1

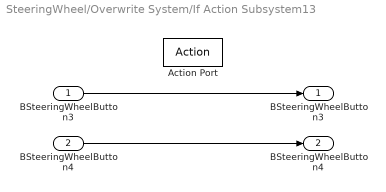
== system SteeringWheel/Overwrite System/If Action Subsystem13 ==
  "BSteeringWheelButton3  " : Inport  OutDataTypeStr=boolean
  "BSteeringWheelButton4  " : Inport  Port=2  OutDataTypeStr=boolean
  Action Port : ActionPort  ActionPortLabel=elseif( u1==12)
  BSteeringWheelButton3 : Outport  OutDataTypeStr=boolean  VectorParamsAs1DForOutWhenUnconnected=off
  BSteeringWheelButton4 : Outport  Port=2  OutDataTypeStr=boolean  VectorParamsAs1DForOutWhenUnconnected=off
  wires:
  "BSteeringWheelButton4  "/1 -> BSteeringWheelButton4/1
  "BSteeringWheelButton3  "/1 -> BSteeringWheelButton3/1

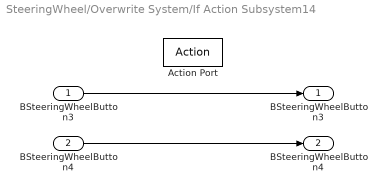
== system SteeringWheel/Overwrite System/If Action Subsystem14 ==
  "BSteeringWheelButton3  " : Inport  OutDataTypeStr=boolean
  "BSteeringWheelButton4  " : Inport  Port=2  OutDataTypeStr=boolean
  Action Port : ActionPort  ActionPortLabel=elseif( u1==14)
  BSteeringWheelButton3 : Outport  OutDataTypeStr=boolean  VectorParamsAs1DForOutWhenUnconnected=off
  BSteeringWheelButton4 : Outport  Port=2  OutDataTypeStr=boolean  VectorParamsAs1DForOutWhenUnconnected=off
  wires:
  "BSteeringWheelButton4  "/1 -> BSteeringWheelButton4/1
  "BSteeringWheelButton3  "/1 -> BSteeringWheelButton3/1

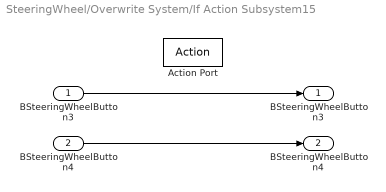
== system SteeringWheel/Overwrite System/If Action Subsystem15 ==
  "BSteeringWheelButton3  " : Inport  OutDataTypeStr=boolean
  "BSteeringWheelButton4  " : Inport  Port=2  OutDataTypeStr=boolean
  Action Port : ActionPort  ActionPortLabel=elseif( u1==15)
  BSteeringWheelButton3 : Outport  OutDataTypeStr=boolean  VectorParamsAs1DForOutWhenUnconnected=off
  BSteeringWheelButton4 : Outport  Port=2  OutDataTypeStr=boolean  VectorParamsAs1DForOutWhenUnconnected=off
  wires:
  "BSteeringWheelButton3  "/1 -> BSteeringWheelButton3/1
  "BSteeringWheelButton4  "/1 -> BSteeringWheelButton4/1

== system SteeringWheel/Overwrite System/If Action Subsystem2 ==
  "BSteeringWheelButton3  " : Inport  OutDataTypeStr=boolean
  "BSteeringWheelButton4  " : Inport  Port=2  OutDataTypeStr=boolean
  Action Port : ActionPort  ActionPortLabel=elseif( u1==3)
  BSteeringWheelButton3 : Outport  OutDataTypeStr=boolean  VectorParamsAs1DForOutWhenUnconnected=off
  BSteeringWheelButton4 : Outport  Port=2  OutDataTypeStr=boolean  VectorParamsAs1DForOutWhenUnconnected=off
  wires:
  "BSteeringWheelButton3  "/1 -> BSteeringWheelButton3/1
  "BSteeringWheelButton4  "/1 -> BSteeringWheelButton4/1

== system SteeringWheel/Overwrite System/If Action Subsystem3 ==
  "BSteeringWheelButton3  " : Inport  OutDataTypeStr=boolean
  "BSteeringWheelButton4  " : Inport  Port=2  OutDataTypeStr=boolean
  Action Port : ActionPort  ActionPortLabel=elseif( u1==4)
  BSteeringWheelButton3 : Outport  OutDataTypeStr=boolean  VectorParamsAs1DForOutWhenUnconnected=off
  BSteeringWheelButton4 : Outport  Port=2  OutDataTypeStr=boolean  VectorParamsAs1DForOutWhenUnconnected=off
  wires:
  "BSteeringWheelButton4  "/1 -> BSteeringWheelButton4/1
  "BSteeringWheelButton3  "/1 -> BSteeringWheelButton3/1

== system SteeringWheel/Overwrite System/If Action Subsystem4 ==
  "BSteeringWheelButton3  " : Inport  OutDataTypeStr=boolean
  "BSteeringWheelButton4  " : Inport  Port=2  OutDataTypeStr=boolean
  Action Port : ActionPort  ActionPortLabel=elseif( u1==5)
  BSteeringWheelButton3 : Outport  OutDataTypeStr=boolean  VectorParamsAs1DForOutWhenUnconnected=off
  BSteeringWheelButton4 : Outport  Port=2  OutDataTypeStr=boolean  VectorParamsAs1DForOutWhenUnconnected=off
  wires:
  "BSteeringWheelButton3  "/1 -> BSteeringWheelButton3/1
  "BSteeringWheelButton4  "/1 -> BSteeringWheelButton4/1

== system SteeringWheel/Overwrite System/If Action Subsystem5 ==
  "BSteeringWheelButton3  " : Inport  OutDataTypeStr=boolean
  "BSteeringWheelButton4  " : Inport  Port=2  OutDataTypeStr=boolean
  Action Port : ActionPort  ActionPortLabel=elseif( u1==6)
  BSteeringWheelButton3 : Outport  OutDataTypeStr=boolean  VectorParamsAs1DForOutWhenUnconnected=off
  BSteeringWheelButton4 : Outport  Port=2  OutDataTypeStr=boolean  VectorParamsAs1DForOutWhenUnconnected=off
  wires:
  "BSteeringWheelButton4  "/1 -> BSteeringWheelButton4/1
  "BSteeringWheelButton3  "/1 -> BSteeringWheelButton3/1

== system SteeringWheel/Overwrite System/If Action Subsystem6 ==
  "BSteeringWheelButton3  " : Inport  OutDataTypeStr=boolean
  "BSteeringWheelButton4  " : Inport  Port=2  OutDataTypeStr=boolean
  Action Port : ActionPort  ActionPortLabel=elseif( u1==7)
  BSteeringWheelButton3 : Outport  OutDataTypeStr=boolean  VectorParamsAs1DForOutWhenUnconnected=off
  BSteeringWheelButton4 : Outport  Port=2  OutDataTypeStr=boolean  VectorParamsAs1DForOutWhenUnconnected=off
  wires:
  "BSteeringWheelButton3  "/1 -> BSteeringWheelButton3/1
  "BSteeringWheelButton4  "/1 -> BSteeringWheelButton4/1

== system SteeringWheel/Overwrite System/If Action Subsystem7 ==
  "BSteeringWheelButton3  " : Inport  OutDataTypeStr=boolean
  "BSteeringWheelButton4  " : Inport  Port=2  OutDataTypeStr=boolean
  Action Port : ActionPort  ActionPortLabel=elseif( u1==8)
  BSteeringWheelButton3 : Outport  OutDataTypeStr=boolean  VectorParamsAs1DForOutWhenUnconnected=off
  BSteeringWheelButton4 : Outport  Port=2  OutDataTypeStr=boolean  VectorParamsAs1DForOutWhenUnconnected=off
  wires:
  "BSteeringWheelButton4  "/1 -> BSteeringWheelButton4/1
  "BSteeringWheelButton3  "/1 -> BSteeringWheelButton3/1

== system SteeringWheel/Overwrite System/If Action Subsystem8 ==
  "BSteeringWheelButton3  " : Inport  OutDataTypeStr=boolean
  "BSteeringWheelButton4  " : Inport  Port=2  OutDataTypeStr=boolean
  Action Port : ActionPort  ActionPortLabel=elseif( u1==9)
  BSteeringWheelButton3 : Outport  OutDataTypeStr=boolean  VectorParamsAs1DForOutWhenUnconnected=off
  BSteeringWheelButton4 : Outport  Port=2  OutDataTypeStr=boolean  VectorParamsAs1DForOutWhenUnconnected=off
  wires:
  "BSteeringWheelButton3  "/1 -> BSteeringWheelButton3/1
  "BSteeringWheelButton4  "/1 -> BSteeringWheelButton4/1

== system SteeringWheel/Overwrite System/If Action Subsystem9 ==
  "BSteeringWheelButton3  " : Inport  OutDataTypeStr=boolean
  "BSteeringWheelButton4  " : Inport  Port=2  OutDataTypeStr=boolean
  Action Port : ActionPort  ActionPortLabel=elseif( u1==10)
  BSteeringWheelButton3 : Outport  OutDataTypeStr=boolean  VectorParamsAs1DForOutWhenUnconnected=off
  BSteeringWheelButton4 : Outport  Port=2  OutDataTypeStr=boolean  VectorParamsAs1DForOutWhenUnconnected=off
  wires:
  "BSteeringWheelButton4  "/1 -> BSteeringWheelButton4/1
  "BSteeringWheelButton3  "/1 -> BSteeringWheelButton3/1

== stateflow chart SteeringWheel/Overwrite System/PEngineBraking ==
  state Map12
    entry:
    PEngineBraking = -1;
  state a
    entry, during:
    PEngineBraking = 0;
  state a1
    entry, during:
    PEngineBraking = 6;
  state a2
    entry, during:
    PEngineBraking = 10;
  state a3
    entry, during:
    PEngineBraking = 14;
  (default) -> Map12
  a -> a1 [order 1] : after(500,tick)
      | [BSteeringWheelButton3 == 1]
  a2 -> a3 [order 2] : after(500,tick)
      | [BSteeringWheelButton3 == 1]
  Map12 -> a [order 1] : after(500,tick)
      | [BSteeringWheelButton3 == 1]
  a1 -> a2 [order 1] : after(500,tick)
      | [BSteeringWheelButton3 == 1]
  a -> Map12 [order 2] : after(500,tick)
      | [BSteeringWheelButton4 ==1]
  a1 -> a [order 2] : after(500,tick)
      | [BSteeringWheelButton4 ==1]
  Map12 -> a3 [order 2] : after(500,tick)
      | [BSteeringWheelButton4 ==1]
  a3 -> Map12 [order 2] : after(500,tick)
      | [BSteeringWheelButton3 == 1]
  a2 -> a1 [order 1] : after(500,tick)
      | [BSteeringWheelButton4 ==1]
  a3 -> a2 [order 1] : after(500,tick)
      | [BSteeringWheelButton4 ==1]
  data: BSteeringWheelButton3 input double; BSteeringWheelButton4 input double; PEngineBraking output double

== stateflow chart SteeringWheel/Overwrite System/PRegenMax ==
  state Map13
    entry:
    PRegenMaxOW = -1;
  state Map12
    entry:
    PRegenMaxOW = 10;
  state Map7
    entry, during:
    PRegenMaxOW = 20;
  state Map8
    entry, during:
    PRegenMaxOW = 30;
  state Map9
    entry, during:
    PRegenMaxOW = 40;
  state Map10
    entry, during:
    PRegenMaxOW = 60;
  state Map14
    entry, during:
    PRegenMaxOW = 80;
  state Map15
    entry, during:
    PRegenMaxOW = 100;
  state Map11
    entry, during:
    PRegenMaxOW = 0;
  Map15 -> Map11 [order 2] : after(500,tick)
      | [BSteeringWheelButton3 == 1]
  Map10 -> Map14 [order 1] : after(500,tick)
      | [BSteeringWheelButton3 == 1]
  Map14 -> Map15 [order 1] : after(500,tick)
      | [BSteeringWheelButton3 == 1]
  Map9 -> Map10 [order 2] : after(500,tick)
      | [BSteeringWheelButton3 == 1]
  Map8 -> Map9 [order 2] : after(500,tick)
      | [BSteeringWheelButton3 == 1]
  Map7 -> Map8 [order 2] : after(500,tick)
      | [BSteeringWheelButton3 == 1]
  (default) -> Map13
  Map12 -> Map7 [order 1] : after(500,tick)
      | [BSteeringWheelButton3 == 1]
  Map13 -> Map12 [order 1] : after(500,tick)
      | [BSteeringWheelButton3 == 1]
  Map13 -> Map11 [order 2] : after(500,tick)
      | [BSteeringWheelButton4 ==1]
  Map11 -> Map13 [order 1] : after(500,tick)
      | [BSteeringWheelButton3 == 1]
  Map7 -> Map12 [order 1] : after(500,tick)
      | [BSteeringWheelButton4 ==1]
  Map8 -> Map7 [order 1] : after(500,tick)
      | [BSteeringWheelButton4 ==1]
  Map9 -> Map8 [order 1] : after(500,tick)
      | [BSteeringWheelButton4 ==1]
  Map10 -> Map9 [order 2] : after(500,tick)
      | [BSteeringWheelButton4 ==1]
  Map14 -> Map10 [order 2] : after(500,tick)
      | [BSteeringWheelButton4 ==1]
  Map15 -> Map14 [order 1] : after(500,tick)
      | [BSteeringWheelButton4 ==1]
  Map11 -> Map15 [order 2] : after(500,tick)
      | [BSteeringWheelButton4 ==1]
  Map12 -> Map13 [order 2] : after(500,tick)
      | [BSteeringWheelButton4 ==1]
  data: BSteeringWheelButton3 input double; BSteeringWheelButton4 input double; PRegenMaxOW output double

== stateflow chart SteeringWheel/Overwrite System/NTCKdSelector  ==
  state Map12
    entry:
    NTCKdSelector = 5;
  state a
    entry, during:
    NTCKdSelector = 4;
  state a2
    entry, during:
    NTCKdSelector = 2;
  state a3
    entry, during:
    NTCKdSelector = 1;
  state a1
    entry, during:
    NTCKdSelector = 3;
  (default) -> a3
  a -> a1 [order 1] : after(500,tick)
      | [BSteeringWheelButton3 == 1]
  a2 -> a3 [order 2] : after(500,tick)
      | [BSteeringWheelButton3 == 1]
  Map12 -> a [order 1] : after(500,tick)
      | [BSteeringWheelButton3 == 1]
  a1 -> a2 [order 1] : after(500,tick)
      | [BSteeringWheelButton3 == 1]
  a -> Map12 [order 2] : after(500,tick)
      | [BSteeringWheelButton4 ==1]
  a1 -> a [order 2] : after(500,tick)
      | [BSteeringWheelButton4 ==1]
  Map12 -> a3 [order 2] : after(500,tick)
      | [BSteeringWheelButton4 ==1]
  a3 -> Map12 [order 2] : after(500,tick)
      | [BSteeringWheelButton3 == 1]
  a2 -> a1 [order 1] : after(500,tick)
      | [BSteeringWheelButton4 ==1]
  a3 -> a2 [order 1] : after(500,tick)
      | [BSteeringWheelButton4 ==1]
  data: BSteeringWheelButton3 input double; BSteeringWheelButton4 input double; NTCKdSelector output double

== stateflow chart SteeringWheel/Overwrite System/NPCKpSelector  ==
  state Map12
    entry:
    NPCKpSelector = 4;
  state a
    entry, during:
    NPCKpSelector = 5;
  state a1
    entry, during:
    NPCKpSelector = 6;
  state a2
    entry, during:
    NPCKpSelector = 1;
  state a3
    entry, during:
    NPCKpSelector = 2;
  state a4
    entry, during:
    NPCKpSelector = 1;
  (default) -> Map12
  a -> a1 [order 1] : after(500,tick)
      | [BSteeringWheelButton3 == 1]
  a2 -> a3 [order 2] : after(500,tick)
      | [BSteeringWheelButton3 == 1]
  a3 -> a4 [order 2] : after(500,tick)
      | [BSteeringWheelButton3 == 1]
  Map12 -> a [order 2] : after(500,tick)
      | [BSteeringWheelButton3 == 1]
  a1 -> a2 [order 1] : after(500,tick)
      | [BSteeringWheelButton3 == 1]
  a -> Map12 [order 2] : after(500,tick)
      | [BSteeringWheelButton4 ==1]
  a1 -> a [order 2] : after(500,tick)
      | [BSteeringWheelButton4 ==1]
  Map12 -> a4 [order 1] : after(500,tick)
      | [BSteeringWheelButton4 ==1]
  a4 -> Map12 [order 2] : after(500,tick)
      | [BSteeringWheelButton3 == 1]
  a2 -> a1 [order 1] : after(500,tick)
      | [BSteeringWheelButton4 ==1]
  a3 -> a2 [order 1] : after(500,tick)
      | [BSteeringWheelButton4 ==1]
  a4 -> a3 [order 1] : after(500,tick)
      | [BSteeringWheelButton4 ==1]
  data: BSteeringWheelButton3 input double; BSteeringWheelButton4 input double; NPCKpSelector output double

== stateflow chart SteeringWheel/Overwrite System/rEngineBrakingSplitOW  ==
  state a4
    entry, during:
    rEngineBrakingSplit = -1;
  state a
    entry, during:
    rEngineBrakingSplit = 0;
  state a2
    entry, during:
    rEngineBrakingSplit = 0.5;
  state a3
    entry, during:
    rEngineBrakingSplit = 1;
  state a1
    entry, during:
    rEngineBrakingSplit = 0.3;
  (default) -> a4
  a2 -> a3 [order 2] : after(500,tick)
      | [BSteeringWheelButton3 == 1]
  a -> a1 [order 1] : after(500,tick)
      | [BSteeringWheelButton3 == 1]
  a4 -> a [order 1] : after(500,tick)
      | [BSteeringWheelButton3 == 1]
  a1 -> a2 [order 1] : after(500,tick)
      | [BSteeringWheelButton3 == 1]
  a4 -> a3 [order 2] : after(500,tick)
      | [BSteeringWheelButton4 ==1]
  a3 -> a4 [order 2] : after(500,tick)
      | [BSteeringWheelButton3 == 1]
  a -> a4 [order 2] : after(500,tick)
      | [BSteeringWheelButton4 ==1]
  a1 -> a [order 2] : after(500,tick)
      | [BSteeringWheelButton4 ==1]
  a2 -> a1 [order 1] : after(500,tick)
      | [BSteeringWheelButton4 ==1]
  a3 -> a2 [order 1] : after(500,tick)
      | [BSteeringWheelButton4 ==1]
  data: BSteeringWheelButton3 input double; BSteeringWheelButton4 input double; rEngineBrakingSplit output double

== stateflow chart SteeringWheel/Overwrite System/BTVOn ==
  state Map12
    entry:
    BTVOnOW = 1;
  state Map13
    entry, during:
    BTVOnOW = -1;
  state Map11
    entry, during:
    BTVOnOW = 0;
  Map13 -> Map12 [order 2] : after(500,tick)
      | [BSteeringWheelButton3 ==1]
  Map11 -> Map12 [order 1] : after(500,tick) [BSteeringWheelButton4==1]
  (default) -> Map13
  Map13 -> Map11 [order 1] : after(500,tick) [BSteeringWheelButton4 ==1]
  Map12 -> Map13 [order 1] : after(500,tick) [BSteeringWheelButton4 ==1]
  Map12 -> Map11 [order 2] : after(500,tick) [BSteeringWheelButton3 ==1]
  Map11 -> Map13 [order 2] : after(500,tick) [BSteeringWheelButton3 ==1]
  data: BSteeringWheelButton3 input double; BSteeringWheelButton4 input double; BTVOnOW output

== stateflow chart SteeringWheel/Overwrite System/BTCOn ==
  state Map12
    entry:
    BTCOnOW = 1;
  state Map11
    entry, during:
    BTCOnOW = 0;
  state Map13
    entry, during:
    BTCOnOW = -1;
  Map13 -> Map12 [order 2] : after(500,tick)
      | [BSteeringWheelButton3 ==1]
  Map11 -> Map12 [order 2] : after(500,tick)
      | [BSteeringWheelButton4 ==1]
  (default) -> Map13
  Map13 -> Map11 [order 1] : after(500,tick)
      | [BSteeringWheelButton4 ==1]
  Map12 -> Map13 [order 2] : after(500,tick)
      | [BSteeringWheelButton4 ==1]
  Map12 -> Map11 [order 1] : after(500,tick)
      | [BSteeringWheelButton3 == 1]
  Map11 -> Map13 [order 1] : after(500,tick)
      | [BSteeringWheelButton3 ==1]
  data: BSteeringWheelButton3 input double; BSteeringWheelButton4 input double; BTCOnOW output

== stateflow chart SteeringWheel/Overwrite System/rTVMultiplier ==
  state Map12
    entry:
    rTVMultiplierOW = 0.1;
  state Map7
    entry, during:
    rTVMultiplierOW = 0.3;
  state Map8
    entry, during:
    rTVMultiplierOW = 0.5;
  state Map9
    entry, during:
    rTVMultiplierOW = 0.7;
  state Map10
    entry, during:
    rTVMultiplierOW = 0;
  state Map11
    entry, during:
    rTVMultiplierOW = 1;
  state Map1
    entry, during:
    rTVMultiplierOW = -1;
  (default) -> Map1
  Map8 -> Map9 [order 2] : after(500,tick)
      | [BSteeringWheelButton3 == 1]
  Map9 -> Map10 [order 2] : after(500,tick)
      | [BSteeringWheelButton3 == 1]
  Map10 -> Map11 [order 2] : after(500,tick)
      | [BSteeringWheelButton3 == 1]
  Map7 -> Map8 [order 2] : after(500,tick)
      | [BSteeringWheelButton3 == 1]
  Map12 -> Map7 [order 1] : after(500,tick)
      | [BSteeringWheelButton3 == 1]
  Map11 -> Map1 [order 2] : after(500,tick)
      | [BSteeringWheelButton3 == 1]
  Map9 -> Map8 [order 1] : after(500,tick)
      | [BSteeringWheelButton4 ==1]
  Map10 -> Map9 [order 1] : after(500,tick)
      | [BSteeringWheelButton4 ==1]
  Map12 -> Map1 [order 2] : after(500,tick)
      | [BSteeringWheelButton4 ==1]
  Map1 -> Map12 [order 1] : after(500,tick)
      | [BSteeringWheelButton3 == 1]
  Map8 -> Map7 [order 1] : after(500,tick)
      | [BSteeringWheelButton4 ==1]
  Map11 -> Map10 [order 1] : after(500,tick)
      | [BSteeringWheelButton4 ==1]
  Map1 -> Map11 [order 2] : after(500,tick)
      | [BSteeringWheelButton4 ==1]
  Map7 -> Map12 [order 1] : after(500,tick)
      | [BSteeringWheelButton4 ==1]
  data: BSteeringWheelButton3 input double; BSteeringWheelButton4 input double; rTVMultiplierOW output double

== stateflow chart SteeringWheel/Overwrite System/BDrivetrainCoolingOn ==
  state Map12
    entry:
    BDrivetrainCoolingOW = 1;
  state Map11
    entry, during:
    BDrivetrainCoolingOW = 0;
  state Map13
    entry, during:
    BDrivetrainCoolingOW = -1;
  Map13 -> Map12 [order 2] : after(500,tick)
      | [BSteeringWheelButton3 ==1]
  Map11 -> Map12 [order 1] : after(500,tick)
      | [BSteeringWheelButton4 == 1]
  (default) -> Map13
  Map13 -> Map11 [order 1] : after(500,tick)
      | [BSteeringWheelButton4 ==1]
  Map12 -> Map13 [order 2] : after(500,tick)
      | [BSteeringWheelButton4 ==1]
  Map12 -> Map11 [order 1] : after(500,tick)
      | [BSteeringWheelButton3 == 1]
  Map11 -> Map13 [order 2] : after(500,tick)
      | [BSteeringWheelButton3 ==1]
  data: BSteeringWheelButton3 input double; BSteeringWheelButton4 input double; BDrivetrainCoolingOW output double

== stateflow chart SteeringWheel/Overwrite System/rGrip ==
  state mode2
    entry, during:
    rGrip = 0.25;
  state mode3
    entry, during:
    rGrip = 0.5;
  state mode4
    entry, during:
    rGrip = 0.75;
  state mode5
    entry, during:
    rGrip = 1;
  mode4 -> mode5 [order 1] : after(500,tick)
      | [BSteeringWheelButton3 == 1]
  mode3 -> mode4 [order 1] : after(500,tick)
      | [BSteeringWheelButton3 == 1]
  mode2 -> mode3 [order 1] : after(500,tick)
      | [BSteeringWheelButton3 == 1]
  (default) -> mode3
  mode2 -> mode5 [order 2] : after(500,tick)
      | [BSteeringWheelButton4 ==1]
  mode5 -> mode2 [order 2] : after(500,tick)
      | [BSteeringWheelButton3 == 1]
  mode3 -> mode2 [order 2] : after(500,tick)
      | [BSteeringWheelButton4 ==1]
  mode4 -> mode3 [order 2] : after(500,tick)
      | [BSteeringWheelButton4 ==1]
  mode5 -> mode4 [order 1] : after(500,tick)
      | [BSteeringWheelButton4 ==1]
  data: BSteeringWheelButton3 input double; BSteeringWheelButton4 input double; rGrip output double
